simulink library "ReceiveFromInputDevice"  (R2016b)
settings: Solver=VariableStepAuto  StartTime=0.0  StopTime=10.0  RelTol=1e-3
libraries: xpcethercatlib x3
settings Model: Creator=Nathan  LastModifiedBy=MARCH

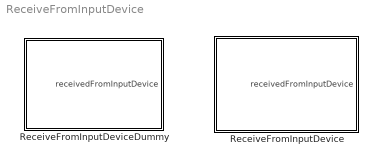
== system ReceiveFromInputDevice ==
  ReceiveFromInputDevice : Subsystem
  ReceiveFromInputDeviceDummy : Subsystem

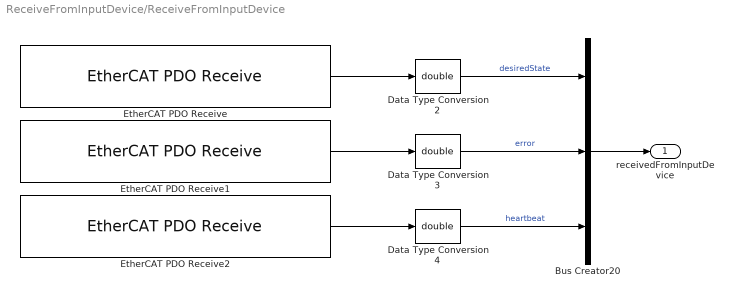
== system ReceiveFromInputDevice/ReceiveFromInputDevice ==
  Bus Creator20 : BusCreator  Inputs=3  OutDataTypeStr=Bus: EtherCATReceivedFromInputDevice  NonVirtualBus=on
  Data Type Conversion2 : DataTypeConversion  OutDataTypeStr=double
  Data Type Conversion3 : DataTypeConversion  OutDataTypeStr=double
  Data Type Conversion4 : DataTypeConversion  OutDataTypeStr=double
  EtherCAT PDO Receive : xpcethercatlib/EtherCAT PDO Receive  Priority=2  sig_name=InputDevice.Inputs.desiredState  sig_offset=720  sig_type=uint8  type_size=8  sig_dim=1  device_id=0  sample_time=0.002000
  EtherCAT PDO Receive1 : xpcethercatlib/EtherCAT PDO Receive  Priority=2  sig_name=InputDevice.Inputs.inputDeviceError  sig_offset=728  sig_type=uint8  type_size=8  sig_dim=1  device_id=0  sample_time=0.002000
  EtherCAT PDO Receive2 : xpcethercatlib/EtherCAT PDO Receive  Priority=2  sig_name=InputDevice.Inputs.heartbeat  sig_offset=2048  sig_type=uint8  type_size=8  sig_dim=1  device_id=0  sample_time=0.002
  receivedFromInputDevice : Outport
  wires:
  EtherCAT PDO Receive1/1 -> Data Type Conversion3/1
  EtherCAT PDO Receive/1 -> Data Type Conversion2/1
  Data Type Conversion2/1 -> Bus Creator20/1  "desiredState"
  Data Type Conversion3/1 -> Bus Creator20/2  "error"
  EtherCAT PDO Receive2/1 -> Data Type Conversion4/1
  Data Type Conversion4/1 -> Bus Creator20/3  "heartbeat"
  Bus Creator20/1 -> receivedFromInputDevice/1

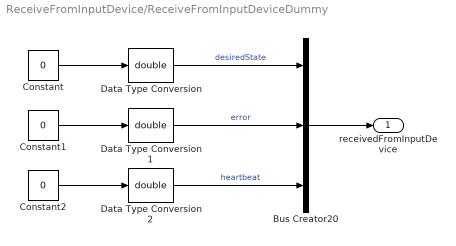
== system ReceiveFromInputDevice/ReceiveFromInputDeviceDummy ==
  Bus Creator20 : BusCreator  Inputs=3  OutDataTypeStr=Bus: EtherCATReceivedFromInputDevice  NonVirtualBus=on
  Constant : Constant  Value=0
  Constant1 : Constant  Value=0
  Constant2 : Constant  Value=0
  Data Type Conversion : DataTypeConversion  OutDataTypeStr=double
  Data Type Conversion1 : DataTypeConversion  OutDataTypeStr=double
  Data Type Conversion2 : DataTypeConversion  OutDataTypeStr=double
  receivedFromInputDevice : Outport
  wires:
  Constant1/1 -> Data Type Conversion1/1
  Constant/1 -> Data Type Conversion/1
  Data Type Conversion/1 -> Bus Creator20/1  "desiredState"
  Data Type Conversion1/1 -> Bus Creator20/2  "error"
  Constant2/1 -> Data Type Conversion2/1
  Data Type Conversion2/1 -> Bus Creator20/3  "heartbeat"
  Bus Creator20/1 -> receivedFromInputDevice/1
